simulink model "general_charger_2 (Jordans MacBook.lan's conflicted copy 2013-12-22)"  (R2013a)
settings: Solver=ode45  StartTime=0  StopTime=2.5  RelTol=1e-3
PreLoadFcn:
  | Ts =5e-6;
values from neighbouring files (symbols this model uses):
  ac_volt = 169    [charger_init.m]    (also in charger_init_simpl.m)
  Cdc = 2e-3    (= 0.002)    [charger_init.m]    (also in charger_init_simpl.m)
  dcAd = dcinvexp*(eye(dcnstates) + (Ts/2)*dcAc)    [charger_init.m]    (also in charger_init_simpl.m)
  dcBd = dcinvexp*dcBc    [charger_init.m]    (also in charger_init_simpl.m)
  dcCd = dcCc*dcinvexp*Ts    [charger_init.m]    (also in charger_init_simpl.m)
  dcDd = dcCc*dcinvexp*dcBc*(Ts/2) + dcDc    [charger_init.m]    (also in charger_init_simpl.m)
  Lin = 1.5e-3    (= 0.0015)    [charger_init.m]    (also in charger_init_simpl.m = 0.001)
  P = 1.92e3    (= 1920)    [charger_init.m]    (also in charger_init_simpl.m)
  Q = 0    [charger_init.m]    (also in charger_init_simpl.m)
  ramp = (dc_volt - Vdcmin)/(acdc_ramp_end_time)    (= 202)    [charger_init.m]    (also in charger_init_simpl.m = (dc_volt - Vdcmin)/(acdc_ramp_end_time))
  switch_Ts = 5e-5    (= 5e-05)    [charger_init.m]    (also in charger_init_simpl.m)
  sys_Ts = 5e-6    (= 5e-06)    [charger_init.m]    (also in charger_init_simpl.m)
  Vdcmin = ac_volt + 10    (= 179)    [charger_init.m]    (also in charger_init_simpl.m)
  voc = 105    [charger_init.m]    (also in charger_init_simpl.m)
undefined symbols (not defined in the file or in its folder): CESR, DiscIntNeverNeededParam, Rin
undefined symbols (not defined in the file): active_power_on, Ad, Bd, Cd, dc_volt, dcdc_iki, dcdc_ikp, dcdc_on, dcdc_vki, dcdc_vkp, Dd, dq_id_ki, dq_id_kp, dq_iq_ki, dq_iq_kp, dq_vdc_ki, dq_vdc_kp, P_ki, P_kp, Q_ki, Q_kp, reactive_power_on
libraries: simulink_extras x165, powerlib x52, simulink x29, powerlib_meascontrol x6
(part 2 of 6)

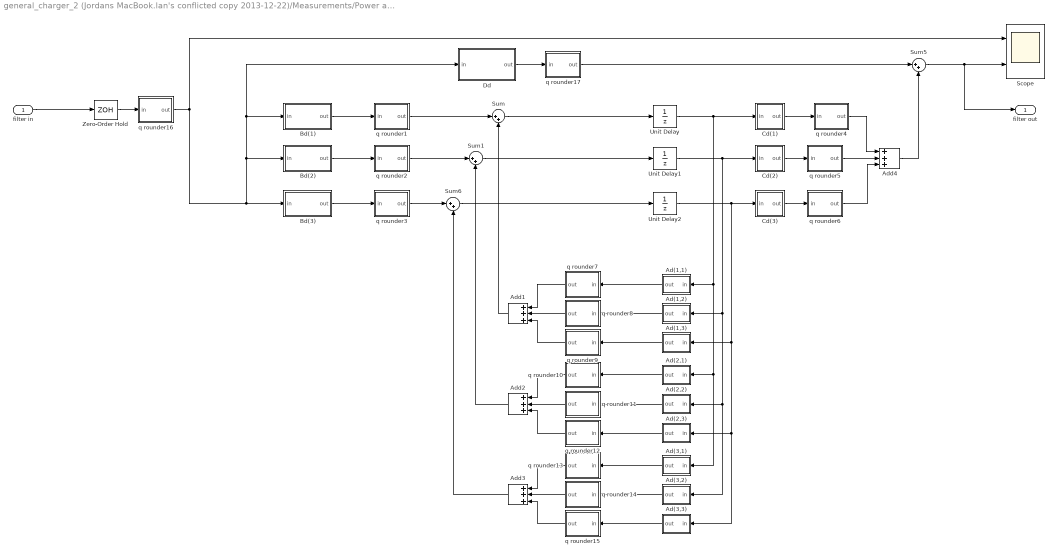
== system general_charger_2 (Jordans MacBook.lan's conflicted copy 2013-12-22)/Measurements/Power and angle calculations/discrete low pass filter1 ==
  filter in : Inport
  Ad(1,1) : Subsystem  mask{variable=Ad(1,1), nQ=29, maxRange=4}
      mask prompts: variable "state-space variable"; nQ "q value"; maxRange "max range"
      mask Display: disp(nQ)
  Ad(1,2) : Subsystem  mask{variable=Ad(1,2), nQ=23, maxRange=256}
      mask prompts: variable "state-space variable"; nQ "q value"; maxRange "max range"
      mask Display: disp(nQ)
  Ad(1,3) : Subsystem  mask{variable=Ad(1,3), nQ=14, maxRange=131072}
      mask prompts: variable "state-space variable"; nQ "q value"; maxRange "max range"
      mask Display: disp(nQ)
  Ad(2,1) : Subsystem  mask{variable=Ad(2,1), nQ=30, maxRange=2}
      mask prompts: variable "state-space variable"; nQ "q value"; maxRange "max range"
      mask Display: disp(nQ)
  Ad(2,2) : Subsystem  mask{variable=Ad(2,2), nQ=29, maxRange=4}
      mask prompts: variable "state-space variable"; nQ "q value"; maxRange "max range"
      mask Display: disp(nQ)
  Ad(2,3) : Subsystem  mask{variable=Ad(2,3), nQ=29, maxRange=4}
      mask prompts: variable "state-space variable"; nQ "q value"; maxRange "max range"
      mask Display: disp(nQ)
  Ad(3,1) : Subsystem  mask{variable=Ad(3,1), nQ=30, maxRange=2}
      mask prompts: variable "state-space variable"; nQ "q value"; maxRange "max range"
      mask Display: disp(nQ)
  Ad(3,2) : Subsystem  mask{variable=Ad(3,2), nQ=30, maxRange=2}
      mask prompts: variable "state-space variable"; nQ "q value"; maxRange "max range"
      mask Display: disp(nQ)
  Ad(3,3) : Subsystem  mask{variable=Ad(3,3), nQ=29, maxRange=4}
      mask prompts: variable "state-space variable"; nQ "q value"; maxRange "max range"
      mask Display: disp(nQ)
  Add{1..4} (4 alike) : Sum  Inputs=+++
  Bd(1) : Subsystem  mask{variable=Bd(1), nQ=29, maxRange=4}
      mask prompts: variable "state-space variable"; nQ "q value"; maxRange "max range"
      mask Display: disp(nQ)
  Bd(2) : Subsystem  mask{variable=Bd(2), nQ=30, maxRange=2}
      mask prompts: variable "state-space variable"; nQ "q value"; maxRange "max range"
      mask Display: disp(nQ)
  Bd(3) : Subsystem  mask{variable=Bd(3), nQ=30, maxRange=2}
      mask prompts: variable "state-space variable"; nQ "q value"; maxRange "max range"
      mask Display: disp(nQ)
  Cd(1) : Subsystem  mask{variable=Cd(1), nQ=30, maxRange=2}
      mask prompts: variable "state-space variable"; nQ "q value"; maxRange "max range"
      mask Display: disp(nQ)
  Cd(2) : Subsystem  mask{variable=Cd(2), nQ=23, maxRange=256}
      mask prompts: variable "state-space variable"; nQ "q value"; maxRange "max range"
      mask Display: disp(nQ)
  Cd(3) : Subsystem  mask{variable=Cd(3), nQ=15, maxRange=65536}
      mask prompts: variable "state-space variable"; nQ "q value"; maxRange "max range"
      mask Display: disp(nQ)
  Dd : Subsystem  mask{variable=Dd, nQ=30, maxRange=2}
      mask prompts: variable "state-space variable"; nQ "q value"; maxRange "max range"
      mask Display: disp(nQ)
  Scope : Scope  NumInputPorts=2
      settings: YMin=-5~-5  YMax=5~5  SaveName=ScopeData11
  Sum{,1,5..6} (4 alike) : Sum  Inputs=|++
  Unit Delay : UnitDelay  SampleTime=5e-5
  Unit Delay1 : UnitDelay  SampleTime=5e-5
  Unit Delay2 : UnitDelay  SampleTime=5e-5
  Zero-Order Hold : ZeroOrderHold  SampleTime=5e-5
  q rounder1 : Subsystem  mask{q=22, range=512}
      mask prompts: q "q value"; range "q range"
      mask Display: disp(q)
  q rounder10 : Subsystem  mask{q=30, range=2}
      mask prompts: q "q value"; range "q range"
      mask Display: disp(q)
  q rounder11 : Subsystem  mask{q=30, range=2}
      mask prompts: q "q value"; range "q range"
      mask Display: disp(q)
  q rounder12 : Subsystem  mask{q=30, range=2}
      mask prompts: q "q value"; range "q range"
      mask Display: disp(q)
  q rounder13 : Subsystem  mask{q=30, range=2}
      mask prompts: q "q value"; range "q range"
      mask Display: disp(q)
  q rounder14 : Subsystem  mask{q=30, range=2}
      mask prompts: q "q value"; range "q range"
      mask Display: disp(q)
  q rounder15 : Subsystem  mask{q=30, range=2}
      mask prompts: q "q value"; range "q range"
      mask Display: disp(q)
  q rounder16 : Subsystem  mask{q=19, range=4096}
      mask prompts: q "q value"; range "q range"
      mask Display: disp(q)
  q rounder17 : Subsystem  mask{q=30, range=2}
      mask prompts: q "q value"; range "q range"
      mask Display: disp(q)
  q rounder2 : Subsystem  mask{q=30, range=2}
      mask prompts: q "q value"; range "q range"
      mask Display: disp(q)
  q rounder3 : Subsystem  mask{q=30, range=2}
      mask prompts: q "q value"; range "q range"
      mask Display: disp(q)
  q rounder4 : Subsystem  mask{q=19, range=4096}
      mask prompts: q "q value"; range "q range"
      mask Display: disp(q)
  q rounder5 : Subsystem  mask{q=19, range=4096}
      mask prompts: q "q value"; range "q range"
      mask Display: disp(q)
  q rounder6 : Subsystem  mask{q=19, range=4096}
      mask prompts: q "q value"; range "q range"
      mask Display: disp(q)
  q rounder7 : Subsystem  mask{q=22, range=512}
      mask prompts: q "q value"; range "q range"
      mask Display: disp(q)
  q rounder8 : Subsystem  mask{q=22, range=512}
      mask prompts: q "q value"; range "q range"
      mask Display: disp(q)
  q rounder9 : Subsystem  mask{q=22, range=512}
      mask prompts: q "q value"; range "q range"
      mask Display: disp(q)
  filter out : Outport
  wires:
  Sum/1 -> Unit Delay/1
  Sum1/1 -> Unit Delay1/1
  Unit Delay/1 -> Ad(3,1)/1(in), Ad(2,1)/1(in), Ad(1,1)/1(in), Cd(1)/1(in)
  Unit Delay1/1 -> Ad(3,2)/1(in), Ad(2,2)/1(in), Ad(1,2)/1(in), Cd(2)/1(in)
  Dd/1(out) -> q rounder17/1(in)
  Sum5/1 -> filter out/1, Scope/2
  Zero-Order Hold/1 -> q rounder16/1(in)
  Sum6/1 -> Unit Delay2/1
  Unit Delay2/1 -> Ad(1,3)/1(in), Ad(3,3)/1(in), Ad(2,3)/1(in), Cd(3)/1(in)
  Ad(1,2)/1(out) -> q rounder8/1(in)
  Ad(1,1)/1(out) -> q rounder7/1(in)
  Ad(2,1)/1(out) -> q rounder10/1(in)
  Ad(2,3)/1(out) -> q rounder12/1(in)
  Ad(2,2)/1(out) -> q rounder11/1(in)
  Ad(3,2)/1(out) -> q rounder14/1(in)
  Ad(3,1)/1(out) -> q rounder13/1(in)
  Ad(3,3)/1(out) -> q rounder15/1(in)
  Add2/1 -> Sum1/2
  Add3/1 -> Sum6/2
  q rounder2/1(out) -> Sum1/1
  q rounder3/1(out) -> Sum6/1
  q rounder4/1(out) -> Add4/1
  q rounder5/1(out) -> Add4/2
  q rounder6/1(out) -> Add4/3
  q rounder7/1(out) -> Add1/1
  q rounder8/1(out) -> Add1/2
  q rounder9/1(out) -> Add1/3
  q rounder10/1(out) -> Add2/1
  q rounder11/1(out) -> Add2/2
  q rounder12/1(out) -> Add2/3
  q rounder13/1(out) -> Add3/1
  q rounder14/1(out) -> Add3/2
  q rounder15/1(out) -> Add3/3
  Bd(1)/1(out) -> q rounder1/1(in)
  Cd(1)/1(out) -> q rounder4/1(in)
  Bd(2)/1(out) -> q rounder2/1(in)
  Bd(3)/1(out) -> q rounder3/1(in)
  Cd(3)/1(out) -> q rounder6/1(in)
  Cd(2)/1(out) -> q rounder5/1(in)
  Ad(1,3)/1(out) -> q rounder9/1(in)
  q rounder16/1(out) -> Scope/1, Bd(3)/1(in), Bd(2)/1(in), Dd/1(in), Bd(1)/1(in)
  q rounder17/1(out) -> Sum5/1
  Add4/1 -> Sum5/2
  Add1/1 -> Sum/2
  q rounder1/1(out) -> Sum/1
  filter in/1 -> Zero-Order Hold/1

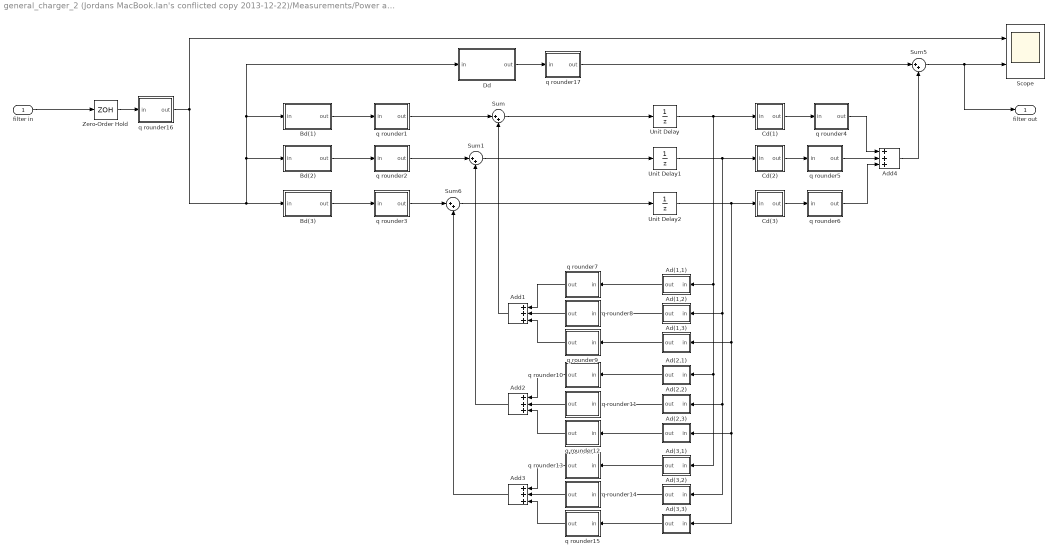
== system general_charger_2 (Jordans MacBook.lan's conflicted copy 2013-12-22)/Measurements/Power and angle calculations/discrete low pass filter2 ==
  filter in : Inport
  Ad(1,1) : Subsystem  mask{variable=Ad(1,1), nQ=29, maxRange=4}
      mask prompts: variable "state-space variable"; nQ "q value"; maxRange "max range"
      mask Display: disp(nQ)
  Ad(1,2) : Subsystem  mask{variable=Ad(1,2), nQ=23, maxRange=256}
      mask prompts: variable "state-space variable"; nQ "q value"; maxRange "max range"
      mask Display: disp(nQ)
  Ad(1,3) : Subsystem  mask{variable=Ad(1,3), nQ=14, maxRange=131072}
      mask prompts: variable "state-space variable"; nQ "q value"; maxRange "max range"
      mask Display: disp(nQ)
  Ad(2,1) : Subsystem  mask{variable=Ad(2,1), nQ=30, maxRange=2}
      mask prompts: variable "state-space variable"; nQ "q value"; maxRange "max range"
      mask Display: disp(nQ)
  Ad(2,2) : Subsystem  mask{variable=Ad(2,2), nQ=29, maxRange=4}
      mask prompts: variable "state-space variable"; nQ "q value"; maxRange "max range"
      mask Display: disp(nQ)
  Ad(2,3) : Subsystem  mask{variable=Ad(2,3), nQ=29, maxRange=4}
      mask prompts: variable "state-space variable"; nQ "q value"; maxRange "max range"
      mask Display: disp(nQ)
  Ad(3,1) : Subsystem  mask{variable=Ad(3,1), nQ=30, maxRange=2}
      mask prompts: variable "state-space variable"; nQ "q value"; maxRange "max range"
      mask Display: disp(nQ)
  Ad(3,2) : Subsystem  mask{variable=Ad(3,2), nQ=30, maxRange=2}
      mask prompts: variable "state-space variable"; nQ "q value"; maxRange "max range"
      mask Display: disp(nQ)
  Ad(3,3) : Subsystem  mask{variable=Ad(3,3), nQ=29, maxRange=4}
      mask prompts: variable "state-space variable"; nQ "q value"; maxRange "max range"
      mask Display: disp(nQ)
  Add{1..4} (4 alike) : Sum  Inputs=+++
  Bd(1) : Subsystem  mask{variable=Bd(1), nQ=29, maxRange=4}
      mask prompts: variable "state-space variable"; nQ "q value"; maxRange "max range"
      mask Display: disp(nQ)
  Bd(2) : Subsystem  mask{variable=Bd(2), nQ=30, maxRange=2}
      mask prompts: variable "state-space variable"; nQ "q value"; maxRange "max range"
      mask Display: disp(nQ)
  Bd(3) : Subsystem  mask{variable=Bd(3), nQ=30, maxRange=2}
      mask prompts: variable "state-space variable"; nQ "q value"; maxRange "max range"
      mask Display: disp(nQ)
  Cd(1) : Subsystem  mask{variable=Cd(1), nQ=30, maxRange=2}
      mask prompts: variable "state-space variable"; nQ "q value"; maxRange "max range"
      mask Display: disp(nQ)
  Cd(2) : Subsystem  mask{variable=Cd(2), nQ=23, maxRange=256}
      mask prompts: variable "state-space variable"; nQ "q value"; maxRange "max range"
      mask Display: disp(nQ)
  Cd(3) : Subsystem  mask{variable=Cd(3), nQ=15, maxRange=65536}
      mask prompts: variable "state-space variable"; nQ "q value"; maxRange "max range"
      mask Display: disp(nQ)
  Dd : Subsystem  mask{variable=Dd, nQ=30, maxRange=2}
      mask prompts: variable "state-space variable"; nQ "q value"; maxRange "max range"
      mask Display: disp(nQ)
  Scope : Scope  NumInputPorts=2
      settings: YMin=-5~-5  YMax=5~5  SaveName=ScopeData11
  Sum{,1,5..6} (4 alike) : Sum  Inputs=|++
  Unit Delay : UnitDelay  SampleTime=5e-5
  Unit Delay1 : UnitDelay  SampleTime=5e-5
  Unit Delay2 : UnitDelay  SampleTime=5e-5
  Zero-Order Hold : ZeroOrderHold  SampleTime=5e-5
  q rounder1 : Subsystem  mask{q=22, range=512}
      mask prompts: q "q value"; range "q range"
      mask Display: disp(q)
  q rounder10 : Subsystem  mask{q=30, range=2}
      mask prompts: q "q value"; range "q range"
      mask Display: disp(q)
  q rounder11 : Subsystem  mask{q=30, range=2}
      mask prompts: q "q value"; range "q range"
      mask Display: disp(q)
  q rounder12 : Subsystem  mask{q=30, range=2}
      mask prompts: q "q value"; range "q range"
      mask Display: disp(q)
  q rounder13 : Subsystem  mask{q=30, range=2}
      mask prompts: q "q value"; range "q range"
      mask Display: disp(q)
  q rounder14 : Subsystem  mask{q=30, range=2}
      mask prompts: q "q value"; range "q range"
      mask Display: disp(q)
  q rounder15 : Subsystem  mask{q=30, range=2}
      mask prompts: q "q value"; range "q range"
      mask Display: disp(q)
  q rounder16 : Subsystem  mask{q=19, range=4096}
      mask prompts: q "q value"; range "q range"
      mask Display: disp(q)
  q rounder17 : Subsystem  mask{q=30, range=2}
      mask prompts: q "q value"; range "q range"
      mask Display: disp(q)
  q rounder2 : Subsystem  mask{q=30, range=2}
      mask prompts: q "q value"; range "q range"
      mask Display: disp(q)
  q rounder3 : Subsystem  mask{q=30, range=2}
      mask prompts: q "q value"; range "q range"
      mask Display: disp(q)
  q rounder4 : Subsystem  mask{q=19, range=4096}
      mask prompts: q "q value"; range "q range"
      mask Display: disp(q)
  q rounder5 : Subsystem  mask{q=19, range=4096}
      mask prompts: q "q value"; range "q range"
      mask Display: disp(q)
  q rounder6 : Subsystem  mask{q=19, range=4096}
      mask prompts: q "q value"; range "q range"
      mask Display: disp(q)
  q rounder7 : Subsystem  mask{q=22, range=512}
      mask prompts: q "q value"; range "q range"
      mask Display: disp(q)
  q rounder8 : Subsystem  mask{q=22, range=512}
      mask prompts: q "q value"; range "q range"
      mask Display: disp(q)
  q rounder9 : Subsystem  mask{q=22, range=512}
      mask prompts: q "q value"; range "q range"
      mask Display: disp(q)
  filter out : Outport
  wires:
  Sum/1 -> Unit Delay/1
  Sum1/1 -> Unit Delay1/1
  Unit Delay/1 -> Ad(3,1)/1(in), Ad(2,1)/1(in), Ad(1,1)/1(in), Cd(1)/1(in)
  Unit Delay1/1 -> Ad(3,2)/1(in), Ad(2,2)/1(in), Ad(1,2)/1(in), Cd(2)/1(in)
  Dd/1(out) -> q rounder17/1(in)
  Sum5/1 -> filter out/1, Scope/2
  Zero-Order Hold/1 -> q rounder16/1(in)
  Sum6/1 -> Unit Delay2/1
  Unit Delay2/1 -> Ad(1,3)/1(in), Ad(3,3)/1(in), Ad(2,3)/1(in), Cd(3)/1(in)
  Ad(1,2)/1(out) -> q rounder8/1(in)
  Ad(1,1)/1(out) -> q rounder7/1(in)
  Ad(2,1)/1(out) -> q rounder10/1(in)
  Ad(2,3)/1(out) -> q rounder12/1(in)
  Ad(2,2)/1(out) -> q rounder11/1(in)
  Ad(3,2)/1(out) -> q rounder14/1(in)
  Ad(3,1)/1(out) -> q rounder13/1(in)
  Ad(3,3)/1(out) -> q rounder15/1(in)
  Add2/1 -> Sum1/2
  Add3/1 -> Sum6/2
  q rounder2/1(out) -> Sum1/1
  q rounder3/1(out) -> Sum6/1
  q rounder4/1(out) -> Add4/1
  q rounder5/1(out) -> Add4/2
  q rounder6/1(out) -> Add4/3
  q rounder7/1(out) -> Add1/1
  q rounder8/1(out) -> Add1/2
  q rounder9/1(out) -> Add1/3
  q rounder10/1(out) -> Add2/1
  q rounder11/1(out) -> Add2/2
  q rounder12/1(out) -> Add2/3
  q rounder13/1(out) -> Add3/1
  q rounder14/1(out) -> Add3/2
  q rounder15/1(out) -> Add3/3
  Bd(1)/1(out) -> q rounder1/1(in)
  Cd(1)/1(out) -> q rounder4/1(in)
  Bd(2)/1(out) -> q rounder2/1(in)
  Bd(3)/1(out) -> q rounder3/1(in)
  Cd(3)/1(out) -> q rounder6/1(in)
  Cd(2)/1(out) -> q rounder5/1(in)
  Ad(1,3)/1(out) -> q rounder9/1(in)
  q rounder16/1(out) -> Scope/1, Bd(3)/1(in), Bd(2)/1(in), Dd/1(in), Bd(1)/1(in)
  q rounder17/1(out) -> Sum5/1
  Add4/1 -> Sum5/2
  Add1/1 -> Sum/2
  q rounder1/1(out) -> Sum/1
  filter in/1 -> Zero-Order Hold/1

== system general_charger_2 (Jordans MacBook.lan's conflicted copy 2013-12-22)/Measurements/THD/RMS1 ==
  ac in : Inport
  Constant1 : Constant  Value=f  SampleTime=Tsss
  Constant2 : Constant  Value=K1  SampleTime=Tsss
  Constant3 : Constant  Value=K2  SampleTime=Tsss
  Delay : Delay  DelayLength=ceil(SpC)  SampleTime=Tsss
  Gain : Gain  Gain=K1  SaturateOnIntegerOverflow=on  OutDataTypeStr=Inherit: Same as input  ParamDataTypeStr=Inherit: Same as input
  Gain1 : Gain  Gain=K2  SaturateOnIntegerOverflow=on  OutDataTypeStr=Inherit: Same as input  ParamDataTypeStr=Inherit: Same as input
  PI3 : Subsystem  mask{ki=1, kp=0, Ts_pi=5e-5, int_sat_up=inf, int_sat_low=-inf, pi_sat_up=inf, pi_sat_low=-inf}
      mask prompts: ki "Integral Gain"; kp "Proportional Gain"; Ts_pi "Sample Time"; int_sat_up "Integral Saturation Upper"; int_sat_low "Integral Saturation Lower"; pi_sat_up "PI Controller Saturation Upper"; pi_sat_low "PI Controller Saturation Lower"
      mask Display: disp('PI')
  Product3 : Product  SaturateOnIntegerOverflow=on  InputSameDT=on  OutDataTypeStr=Inherit: Same as first input
  Product4 : Product  SaturateOnIntegerOverflow=on  InputSameDT=on  OutDataTypeStr=Inherit: Same as first input
  Saturation : Saturate  UpperLimit=inf  LowerLimit=0
  Scope1 : Scope  NumInputPorts=3
      settings: ShowLegends=on  TimeRange=1  YMin=0~-5~-5  YMax=32.5~5~5  SaveName=is_vs_7  MaxDataPoints=50000
  Scope2 : Scope  NumInputPorts=3
      settings: ShowLegends=on  TimeRange=1  YMin=0~-5~-5  YMax=32.5~5~5  SaveName=is_vs_  MaxDataPoints=50000
  Scope3 : Scope  NumInputPorts=3
      settings: ShowLegends=on  TimeRange=1  YMin=0~-5~-5  YMax=32.5~5~5  SaveName=is_vs_8  MaxDataPoints=50000
  Sqrt : Sqrt  SaturateOnIntegerOverflow=on
  Sum1 : Sum  Inputs=+-  SaturateOnIntegerOverflow=on  InputSameDT=on  OutDataTypeStr=Inherit: Same as first input
  Sum2 : Sum  Inputs=-+  SaturateOnIntegerOverflow=on  InputSameDT=on  OutDataTypeStr=Inherit: Same as first input
  Sum3 : Sum  SaturateOnIntegerOverflow=on  InputSameDT=on  OutDataTypeStr=Inherit: Same as first input
  Unit Delay : UnitDelay  SampleTime=Tsss
  rms out : Outport
  wires:
  Sum2/1 -> Product4/1
  Constant1/1 -> Product4/2
  Delay/1 -> Scope1/2, Sum2/1
  ac in/1 -> Product3/2, Product3/1
  Product3/1 -> Gain1/1, Unit Delay/1, PI3/1(in)
  PI3/1(out) -> Scope1/1, Sum2/2, Delay/1
  Sqrt/1 -> rms out/1
  Gain1/1 -> Scope2/1, Sum1/1
  Unit Delay/1 -> Gain/1
  Gain/1 -> Scope2/2, Sum1/2
  Product4/1 -> Sum3/1
  Sum3/1 -> Saturation/1
  Sum1/1 -> Scope2/3, Sum3/2  "Correction"
  Saturation/1 -> Sqrt/1
  Constant2/1 -> Scope3/1
  Constant3/1 -> Scope3/2

== system general_charger_2 (Jordans MacBook.lan's conflicted copy 2013-12-22)/Measurements/THD/RMS2 ==
  ac in : Inport
  Constant1 : Constant  Value=f  SampleTime=Tsss
  Constant2 : Constant  Value=K1  SampleTime=Tsss
  Constant3 : Constant  Value=K2  SampleTime=Tsss
  Delay : Delay  DelayLength=ceil(SpC)  SampleTime=Tsss
  Gain : Gain  Gain=K1  SaturateOnIntegerOverflow=on  OutDataTypeStr=Inherit: Same as input  ParamDataTypeStr=Inherit: Same as input
  Gain1 : Gain  Gain=K2  SaturateOnIntegerOverflow=on  OutDataTypeStr=Inherit: Same as input  ParamDataTypeStr=Inherit: Same as input
  PI3 : Subsystem  mask{ki=1, kp=0, Ts_pi=5e-5, int_sat_up=inf, int_sat_low=-inf, pi_sat_up=inf, pi_sat_low=-inf}
      mask prompts: ki "Integral Gain"; kp "Proportional Gain"; Ts_pi "Sample Time"; int_sat_up "Integral Saturation Upper"; int_sat_low "Integral Saturation Lower"; pi_sat_up "PI Controller Saturation Upper"; pi_sat_low "PI Controller Saturation Lower"
      mask Display: disp('PI')
  Product3 : Product  SaturateOnIntegerOverflow=on  InputSameDT=on  OutDataTypeStr=Inherit: Same as first input
  Product4 : Product  SaturateOnIntegerOverflow=on  InputSameDT=on  OutDataTypeStr=Inherit: Same as first input
  Saturation : Saturate  UpperLimit=inf  LowerLimit=0
  Scope1 : Scope  NumInputPorts=3
      settings: ShowLegends=on  TimeRange=1  YMin=0~-5~-5  YMax=32.5~5~5  SaveName=is_vs_7  MaxDataPoints=50000
  Scope2 : Scope  NumInputPorts=3
      settings: ShowLegends=on  TimeRange=1  YMin=0~-5~-5  YMax=32.5~5~5  SaveName=is_vs_  MaxDataPoints=50000
  Scope3 : Scope  NumInputPorts=3
      settings: ShowLegends=on  TimeRange=1  YMin=0~-5~-5  YMax=32.5~5~5  SaveName=is_vs_8  MaxDataPoints=50000
  Sqrt : Sqrt  SaturateOnIntegerOverflow=on
  Sum1 : Sum  Inputs=+-  SaturateOnIntegerOverflow=on  InputSameDT=on  OutDataTypeStr=Inherit: Same as first input
  Sum2 : Sum  Inputs=-+  SaturateOnIntegerOverflow=on  InputSameDT=on  OutDataTypeStr=Inherit: Same as first input
  Sum3 : Sum  SaturateOnIntegerOverflow=on  InputSameDT=on  OutDataTypeStr=Inherit: Same as first input
  Unit Delay : UnitDelay  SampleTime=Tsss
  rms out : Outport
  wires:
  Sum2/1 -> Product4/1
  Constant1/1 -> Product4/2
  Delay/1 -> Scope1/2, Sum2/1
  ac in/1 -> Product3/2, Product3/1
  Product3/1 -> Gain1/1, Unit Delay/1, PI3/1(in)
  PI3/1(out) -> Scope1/1, Sum2/2, Delay/1
  Sqrt/1 -> rms out/1
  Gain1/1 -> Scope2/1, Sum1/1
  Unit Delay/1 -> Gain/1
  Gain/1 -> Scope2/2, Sum1/2
  Product4/1 -> Sum3/1
  Sum3/1 -> Saturation/1
  Sum1/1 -> Scope2/3, Sum3/2  "Correction"
  Saturation/1 -> Sqrt/1
  Constant2/1 -> Scope3/1
  Constant3/1 -> Scope3/2

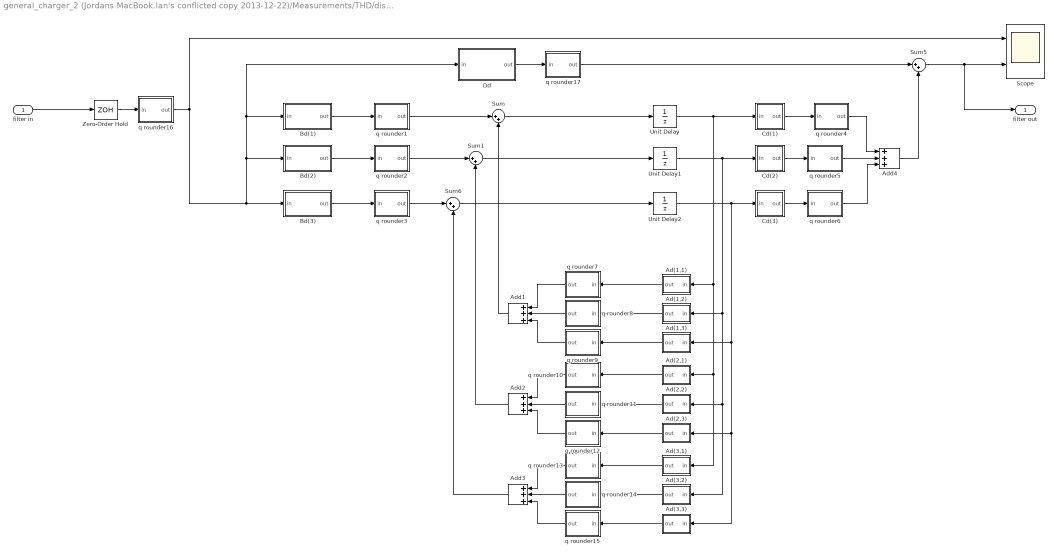
== system general_charger_2 (Jordans MacBook.lan's conflicted copy 2013-12-22)/Measurements/THD/discrete low pass filter1 ==
  filter in : Inport
  Ad(1,1) : Subsystem  mask{variable=Ad(1,1), nQ=29, maxRange=4}
      mask prompts: variable "state-space variable"; nQ "q value"; maxRange "max range"
      mask Display: disp(nQ)
  Ad(1,2) : Subsystem  mask{variable=Ad(1,2), nQ=23, maxRange=256}
      mask prompts: variable "state-space variable"; nQ "q value"; maxRange "max range"
      mask Display: disp(nQ)
  Ad(1,3) : Subsystem  mask{variable=Ad(1,3), nQ=14, maxRange=131072}
      mask prompts: variable "state-space variable"; nQ "q value"; maxRange "max range"
      mask Display: disp(nQ)
  Ad(2,1) : Subsystem  mask{variable=Ad(2,1), nQ=30, maxRange=2}
      mask prompts: variable "state-space variable"; nQ "q value"; maxRange "max range"
      mask Display: disp(nQ)
  Ad(2,2) : Subsystem  mask{variable=Ad(2,2), nQ=29, maxRange=4}
      mask prompts: variable "state-space variable"; nQ "q value"; maxRange "max range"
      mask Display: disp(nQ)
  Ad(2,3) : Subsystem  mask{variable=Ad(2,3), nQ=29, maxRange=4}
      mask prompts: variable "state-space variable"; nQ "q value"; maxRange "max range"
      mask Display: disp(nQ)
  Ad(3,1) : Subsystem  mask{variable=Ad(3,1), nQ=30, maxRange=2}
      mask prompts: variable "state-space variable"; nQ "q value"; maxRange "max range"
      mask Display: disp(nQ)
  Ad(3,2) : Subsystem  mask{variable=Ad(3,2), nQ=30, maxRange=2}
      mask prompts: variable "state-space variable"; nQ "q value"; maxRange "max range"
      mask Display: disp(nQ)
  Ad(3,3) : Subsystem  mask{variable=Ad(3,3), nQ=29, maxRange=4}
      mask prompts: variable "state-space variable"; nQ "q value"; maxRange "max range"
      mask Display: disp(nQ)
  Add{1..4} (4 alike) : Sum  Inputs=+++
  Bd(1) : Subsystem  mask{variable=Bd(1), nQ=29, maxRange=4}
      mask prompts: variable "state-space variable"; nQ "q value"; maxRange "max range"
      mask Display: disp(nQ)
  Bd(2) : Subsystem  mask{variable=Bd(2), nQ=30, maxRange=2}
      mask prompts: variable "state-space variable"; nQ "q value"; maxRange "max range"
      mask Display: disp(nQ)
  Bd(3) : Subsystem  mask{variable=Bd(3), nQ=30, maxRange=2}
      mask prompts: variable "state-space variable"; nQ "q value"; maxRange "max range"
      mask Display: disp(nQ)
  Cd(1) : Subsystem  mask{variable=Cd(1), nQ=30, maxRange=2}
      mask prompts: variable "state-space variable"; nQ "q value"; maxRange "max range"
      mask Display: disp(nQ)
  Cd(2) : Subsystem  mask{variable=Cd(2), nQ=23, maxRange=256}
      mask prompts: variable "state-space variable"; nQ "q value"; maxRange "max range"
      mask Display: disp(nQ)
  Cd(3) : Subsystem  mask{variable=Cd(3), nQ=15, maxRange=65536}
      mask prompts: variable "state-space variable"; nQ "q value"; maxRange "max range"
      mask Display: disp(nQ)
  Dd : Subsystem  mask{variable=Dd, nQ=30, maxRange=2}
      mask prompts: variable "state-space variable"; nQ "q value"; maxRange "max range"
      mask Display: disp(nQ)
  Scope : Scope  NumInputPorts=2
      settings: YMin=-5~-5  YMax=5~5  SaveName=ScopeData11
  Sum{,1,5..6} (4 alike) : Sum  Inputs=|++
  Unit Delay : UnitDelay  SampleTime=5e-5
  Unit Delay1 : UnitDelay  SampleTime=5e-5
  Unit Delay2 : UnitDelay  SampleTime=5e-5
  Zero-Order Hold : ZeroOrderHold  SampleTime=5e-5
  q rounder1 : Subsystem  mask{q=22, range=512}
      mask prompts: q "q value"; range "q range"
      mask Display: disp(q)
  q rounder10 : Subsystem  mask{q=30, range=2}
      mask prompts: q "q value"; range "q range"
      mask Display: disp(q)
  q rounder11 : Subsystem  mask{q=30, range=2}
      mask prompts: q "q value"; range "q range"
      mask Display: disp(q)
  q rounder12 : Subsystem  mask{q=30, range=2}
      mask prompts: q "q value"; range "q range"
      mask Display: disp(q)
  q rounder13 : Subsystem  mask{q=30, range=2}
      mask prompts: q "q value"; range "q range"
      mask Display: disp(q)
  q rounder14 : Subsystem  mask{q=30, range=2}
      mask prompts: q "q value"; range "q range"
      mask Display: disp(q)
  q rounder15 : Subsystem  mask{q=30, range=2}
      mask prompts: q "q value"; range "q range"
      mask Display: disp(q)
  q rounder16 : Subsystem  mask{q=19, range=4096}
      mask prompts: q "q value"; range "q range"
      mask Display: disp(q)
  q rounder17 : Subsystem  mask{q=30, range=2}
      mask prompts: q "q value"; range "q range"
      mask Display: disp(q)
  q rounder2 : Subsystem  mask{q=30, range=2}
      mask prompts: q "q value"; range "q range"
      mask Display: disp(q)
  q rounder3 : Subsystem  mask{q=30, range=2}
      mask prompts: q "q value"; range "q range"
      mask Display: disp(q)
  q rounder4 : Subsystem  mask{q=19, range=4096}
      mask prompts: q "q value"; range "q range"
      mask Display: disp(q)
  q rounder5 : Subsystem  mask{q=19, range=4096}
      mask prompts: q "q value"; range "q range"
      mask Display: disp(q)
  q rounder6 : Subsystem  mask{q=19, range=4096}
      mask prompts: q "q value"; range "q range"
      mask Display: disp(q)
  q rounder7 : Subsystem  mask{q=22, range=512}
      mask prompts: q "q value"; range "q range"
      mask Display: disp(q)
  q rounder8 : Subsystem  mask{q=22, range=512}
      mask prompts: q "q value"; range "q range"
      mask Display: disp(q)
  q rounder9 : Subsystem  mask{q=22, range=512}
      mask prompts: q "q value"; range "q range"
      mask Display: disp(q)
  filter out : Outport
  wires:
  Sum/1 -> Unit Delay/1
  Sum1/1 -> Unit Delay1/1
  Unit Delay/1 -> Ad(3,1)/1(in), Ad(2,1)/1(in), Ad(1,1)/1(in), Cd(1)/1(in)
  Unit Delay1/1 -> Ad(3,2)/1(in), Ad(2,2)/1(in), Ad(1,2)/1(in), Cd(2)/1(in)
  Dd/1(out) -> q rounder17/1(in)
  Sum5/1 -> filter out/1, Scope/2
  Zero-Order Hold/1 -> q rounder16/1(in)
  Sum6/1 -> Unit Delay2/1
  Unit Delay2/1 -> Ad(1,3)/1(in), Ad(3,3)/1(in), Ad(2,3)/1(in), Cd(3)/1(in)
  Ad(1,2)/1(out) -> q rounder8/1(in)
  Ad(1,1)/1(out) -> q rounder7/1(in)
  Ad(2,1)/1(out) -> q rounder10/1(in)
  Ad(2,3)/1(out) -> q rounder12/1(in)
  Ad(2,2)/1(out) -> q rounder11/1(in)
  Ad(3,2)/1(out) -> q rounder14/1(in)
  Ad(3,1)/1(out) -> q rounder13/1(in)
  Ad(3,3)/1(out) -> q rounder15/1(in)
  Add2/1 -> Sum1/2
  Add3/1 -> Sum6/2
  q rounder2/1(out) -> Sum1/1
  q rounder3/1(out) -> Sum6/1
  q rounder4/1(out) -> Add4/1
  q rounder5/1(out) -> Add4/2
  q rounder6/1(out) -> Add4/3
  q rounder7/1(out) -> Add1/1
  q rounder8/1(out) -> Add1/2
  q rounder9/1(out) -> Add1/3
  q rounder10/1(out) -> Add2/1
  q rounder11/1(out) -> Add2/2
  q rounder12/1(out) -> Add2/3
  q rounder13/1(out) -> Add3/1
  q rounder14/1(out) -> Add3/2
  q rounder15/1(out) -> Add3/3
  Bd(1)/1(out) -> q rounder1/1(in)
  Cd(1)/1(out) -> q rounder4/1(in)
  Bd(2)/1(out) -> q rounder2/1(in)
  Bd(3)/1(out) -> q rounder3/1(in)
  Cd(3)/1(out) -> q rounder6/1(in)
  Cd(2)/1(out) -> q rounder5/1(in)
  Ad(1,3)/1(out) -> q rounder9/1(in)
  q rounder16/1(out) -> Scope/1, Bd(3)/1(in), Bd(2)/1(in), Dd/1(in), Bd(1)/1(in)
  q rounder17/1(out) -> Sum5/1
  Add4/1 -> Sum5/2
  Add1/1 -> Sum/2
  q rounder1/1(out) -> Sum/1
  filter in/1 -> Zero-Order Hold/1

== system general_charger_2 (Jordans MacBook.lan's conflicted copy 2013-12-22)/Measurements/discrete low pass filter1/Ad(1,1) ==
  in : Inport
  Constant1 : Constant  Value=variable
  Product1 : Product
  q rounder16 : Subsystem  mask{q=nQ, range=maxRange}
      mask prompts: q "q value"; range "q range"
  out : Outport
  wires:
  q rounder16/1(out) -> Product1/1
  Constant1/1 -> q rounder16/1(in)
  Product1/1 -> out/1
  in/1 -> Product1/2

== system general_charger_2 (Jordans MacBook.lan's conflicted copy 2013-12-22)/Measurements/discrete low pass filter1/Ad(1,2) ==
  in : Inport
  Constant1 : Constant  Value=variable
  Product1 : Product
  q rounder16 : Subsystem  mask{q=nQ, range=maxRange}
      mask prompts: q "q value"; range "q range"
  out : Outport
  wires:
  q rounder16/1(out) -> Product1/1
  Constant1/1 -> q rounder16/1(in)
  Product1/1 -> out/1
  in/1 -> Product1/2

== system general_charger_2 (Jordans MacBook.lan's conflicted copy 2013-12-22)/Measurements/discrete low pass filter1/Ad(1,3) ==
  in : Inport
  Constant1 : Constant  Value=variable
  Product1 : Product
  Scope1 : Scope  NumInputPorts=2
      settings: YMin=-5~-5  YMax=5~5
  q rounder16 : Subsystem  mask{q=nQ, range=maxRange}
      mask prompts: q "q value"; range "q range"
  out : Outport
  wires:
  q rounder16/1(out) -> Product1/1, Scope1/2
  Constant1/1 -> Scope1/1, q rounder16/1(in)
  Product1/1 -> out/1
  in/1 -> Product1/2

== system general_charger_2 (Jordans MacBook.lan's conflicted copy 2013-12-22)/Measurements/discrete low pass filter1/Ad(2,1) ==
  in : Inport
  Constant1 : Constant  Value=variable
  Product1 : Product
  Scope1 : Scope  NumInputPorts=2
      settings: YMin=-5~-5  YMax=5~5
  q rounder16 : Subsystem  mask{q=nQ, range=maxRange}
      mask prompts: q "q value"; range "q range"
  out : Outport
  wires:
  q rounder16/1(out) -> Product1/1, Scope1/2
  Constant1/1 -> Scope1/1, q rounder16/1(in)
  Product1/1 -> out/1
  in/1 -> Product1/2

== system general_charger_2 (Jordans MacBook.lan's conflicted copy 2013-12-22)/Measurements/discrete low pass filter1/Ad(2,2) ==
  in : Inport
  Constant1 : Constant  Value=variable
  Product1 : Product
  Scope1 : Scope  NumInputPorts=2
      settings: YMin=-5~-5  YMax=5~5
  q rounder16 : Subsystem  mask{q=nQ, range=maxRange}
      mask prompts: q "q value"; range "q range"
  out : Outport
  wires:
  q rounder16/1(out) -> Product1/1, Scope1/2
  Constant1/1 -> Scope1/1, q rounder16/1(in)
  Product1/1 -> out/1
  in/1 -> Product1/2

== system general_charger_2 (Jordans MacBook.lan's conflicted copy 2013-12-22)/Measurements/discrete low pass filter1/Ad(2,3) ==
  in : Inport
  Constant1 : Constant  Value=variable
  Product1 : Product
  Scope1 : Scope  NumInputPorts=2
      settings: YMin=-5~-5  YMax=5~5
  q rounder16 : Subsystem  mask{q=nQ, range=maxRange}
      mask prompts: q "q value"; range "q range"
  out : Outport
  wires:
  q rounder16/1(out) -> Product1/1, Scope1/2
  Constant1/1 -> Scope1/1, q rounder16/1(in)
  Product1/1 -> out/1
  in/1 -> Product1/2

== system general_charger_2 (Jordans MacBook.lan's conflicted copy 2013-12-22)/Measurements/discrete low pass filter1/Ad(3,1) ==
  in : Inport
  Constant1 : Constant  Value=variable
  Product1 : Product
  Scope1 : Scope  NumInputPorts=2
      settings: YMin=-5~-5  YMax=5~5
  q rounder16 : Subsystem  mask{q=nQ, range=maxRange}
      mask prompts: q "q value"; range "q range"
  out : Outport
  wires:
  q rounder16/1(out) -> Product1/1, Scope1/2
  Constant1/1 -> Scope1/1, q rounder16/1(in)
  Product1/1 -> out/1
  in/1 -> Product1/2

== system general_charger_2 (Jordans MacBook.lan's conflicted copy 2013-12-22)/Measurements/discrete low pass filter1/Ad(3,2) ==
  in : Inport
  Constant1 : Constant  Value=variable
  Product1 : Product
  Scope1 : Scope  NumInputPorts=2
      settings: YMin=-5~-5  YMax=5~5
  q rounder16 : Subsystem  mask{q=nQ, range=maxRange}
      mask prompts: q "q value"; range "q range"
  out : Outport
  wires:
  q rounder16/1(out) -> Product1/1, Scope1/2
  Constant1/1 -> Scope1/1, q rounder16/1(in)
  Product1/1 -> out/1
  in/1 -> Product1/2

== system general_charger_2 (Jordans MacBook.lan's conflicted copy 2013-12-22)/Measurements/discrete low pass filter1/Ad(3,3) ==
  in : Inport
  Constant1 : Constant  Value=variable
  Product1 : Product
  Scope1 : Scope  NumInputPorts=2
      settings: YMin=-5~-5  YMax=5~5
  q rounder16 : Subsystem  mask{q=nQ, range=maxRange}
      mask prompts: q "q value"; range "q range"
  out : Outport
  wires:
  q rounder16/1(out) -> Product1/1, Scope1/2
  Constant1/1 -> Scope1/1, q rounder16/1(in)
  Product1/1 -> out/1
  in/1 -> Product1/2

== system general_charger_2 (Jordans MacBook.lan's conflicted copy 2013-12-22)/Measurements/discrete low pass filter1/Bd(1) ==
  in : Inport
  Constant1 : Constant  Value=variable
  Product1 : Product
  q rounder16 : Subsystem  mask{q=nQ, range=maxRange}
      mask prompts: q "q value"; range "q range"
  out : Outport
  wires:
  q rounder16/1(out) -> Product1/1
  Constant1/1 -> q rounder16/1(in)
  Product1/1 -> out/1
  in/1 -> Product1/2

== system general_charger_2 (Jordans MacBook.lan's conflicted copy 2013-12-22)/Measurements/discrete low pass filter1/Bd(2) ==
  in : Inport
  Constant1 : Constant  Value=variable
  Product1 : Product
  q rounder16 : Subsystem  mask{q=nQ, range=maxRange}
      mask prompts: q "q value"; range "q range"
  out : Outport
  wires:
  q rounder16/1(out) -> Product1/1
  Constant1/1 -> q rounder16/1(in)
  Product1/1 -> out/1
  in/1 -> Product1/2

== system general_charger_2 (Jordans MacBook.lan's conflicted copy 2013-12-22)/Measurements/discrete low pass filter1/Bd(3) ==
  in : Inport
  Constant1 : Constant  Value=variable
  Product1 : Product
  q rounder16 : Subsystem  mask{q=nQ, range=maxRange}
      mask prompts: q "q value"; range "q range"
  out : Outport
  wires:
  q rounder16/1(out) -> Product1/1
  Constant1/1 -> q rounder16/1(in)
  Product1/1 -> out/1
  in/1 -> Product1/2

== system general_charger_2 (Jordans MacBook.lan's conflicted copy 2013-12-22)/Measurements/discrete low pass filter1/Cd(1) ==
  in : Inport
  Constant1 : Constant  Value=variable
  Product1 : Product
  q rounder16 : Subsystem  mask{q=nQ, range=maxRange}
      mask prompts: q "q value"; range "q range"
  out : Outport
  wires:
  q rounder16/1(out) -> Product1/1
  Constant1/1 -> q rounder16/1(in)
  Product1/1 -> out/1
  in/1 -> Product1/2

== system general_charger_2 (Jordans MacBook.lan's conflicted copy 2013-12-22)/Measurements/discrete low pass filter1/Cd(2) ==
  in : Inport
  Constant1 : Constant  Value=variable
  Product1 : Product
  q rounder16 : Subsystem  mask{q=nQ, range=maxRange}
      mask prompts: q "q value"; range "q range"
  out : Outport
  wires:
  q rounder16/1(out) -> Product1/1
  Constant1/1 -> q rounder16/1(in)
  Product1/1 -> out/1
  in/1 -> Product1/2

== system general_charger_2 (Jordans MacBook.lan's conflicted copy 2013-12-22)/Measurements/discrete low pass filter1/Cd(3) ==
  in : Inport
  Constant1 : Constant  Value=variable
  Product1 : Product
  q rounder16 : Subsystem  mask{q=nQ, range=maxRange}
      mask prompts: q "q value"; range "q range"
  out : Outport
  wires:
  q rounder16/1(out) -> Product1/1
  Constant1/1 -> q rounder16/1(in)
  Product1/1 -> out/1
  in/1 -> Product1/2

== system general_charger_2 (Jordans MacBook.lan's conflicted copy 2013-12-22)/Measurements/discrete low pass filter1/Dd ==
  in : Inport
  Constant1 : Constant  Value=variable
  Product1 : Product
  Scope1 : Scope  NumInputPorts=2
      settings: YMin=-5~-5  YMax=5~5
  q rounder16 : Subsystem  mask{q=nQ, range=maxRange}
      mask prompts: q "q value"; range "q range"
  out : Outport
  wires:
  q rounder16/1(out) -> Product1/1, Scope1/2
  Constant1/1 -> Scope1/1, q rounder16/1(in)
  Product1/1 -> out/1
  in/1 -> Product1/2

== system general_charger_2 (Jordans MacBook.lan's conflicted copy 2013-12-22)/Measurements/discrete low pass filter1/q rounder1 ==
  in : Inport
  Gain9 : Gain  Gain=2^-q
  Idealized ADC quantizer : simulink_extras/Additional Discrete/Idealized ADC quantizer  NumberOfConverterBits=32  Vmin=-range  Vmax=range  OutputDataType=double  OutputNegativeValues=on
  out : Outport
  wires:
  in/1 -> Idealized ADC quantizer/1
  Idealized ADC quantizer/1 -> Gain9/1
  Gain9/1 -> out/1

== system general_charger_2 (Jordans MacBook.lan's conflicted copy 2013-12-22)/Measurements/discrete low pass filter1/q rounder10 ==
  in : Inport
  Gain9 : Gain  Gain=2^-q
  Idealized ADC quantizer : simulink_extras/Additional Discrete/Idealized ADC quantizer  NumberOfConverterBits=32  Vmin=-range  Vmax=range  OutputDataType=double  OutputNegativeValues=on
  out : Outport
  wires:
  in/1 -> Idealized ADC quantizer/1
  Idealized ADC quantizer/1 -> Gain9/1
  Gain9/1 -> out/1

== system general_charger_2 (Jordans MacBook.lan's conflicted copy 2013-12-22)/Measurements/discrete low pass filter1/q rounder11 ==
  in : Inport
  Gain9 : Gain  Gain=2^-q
  Idealized ADC quantizer : simulink_extras/Additional Discrete/Idealized ADC quantizer  NumberOfConverterBits=32  Vmin=-range  Vmax=range  OutputDataType=double  OutputNegativeValues=on
  out : Outport
  wires:
  in/1 -> Idealized ADC quantizer/1
  Idealized ADC quantizer/1 -> Gain9/1
  Gain9/1 -> out/1

== system general_charger_2 (Jordans MacBook.lan's conflicted copy 2013-12-22)/Measurements/discrete low pass filter1/q rounder12 ==
  in : Inport
  Gain9 : Gain  Gain=2^-q
  Idealized ADC quantizer : simulink_extras/Additional Discrete/Idealized ADC quantizer  NumberOfConverterBits=32  Vmin=-range  Vmax=range  OutputDataType=double  OutputNegativeValues=on
  out : Outport
  wires:
  in/1 -> Idealized ADC quantizer/1
  Idealized ADC quantizer/1 -> Gain9/1
  Gain9/1 -> out/1

== system general_charger_2 (Jordans MacBook.lan's conflicted copy 2013-12-22)/Measurements/discrete low pass filter1/q rounder13 ==
  in : Inport
  Gain9 : Gain  Gain=2^-q
  Idealized ADC quantizer : simulink_extras/Additional Discrete/Idealized ADC quantizer  NumberOfConverterBits=32  Vmin=-range  Vmax=range  OutputDataType=double  OutputNegativeValues=on
  out : Outport
  wires:
  in/1 -> Idealized ADC quantizer/1
  Idealized ADC quantizer/1 -> Gain9/1
  Gain9/1 -> out/1

== system general_charger_2 (Jordans MacBook.lan's conflicted copy 2013-12-22)/Measurements/discrete low pass filter1/q rounder14 ==
  in : Inport
  Gain9 : Gain  Gain=2^-q
  Idealized ADC quantizer : simulink_extras/Additional Discrete/Idealized ADC quantizer  NumberOfConverterBits=32  Vmin=-range  Vmax=range  OutputDataType=double  OutputNegativeValues=on
  out : Outport
  wires:
  in/1 -> Idealized ADC quantizer/1
  Idealized ADC quantizer/1 -> Gain9/1
  Gain9/1 -> out/1

== system general_charger_2 (Jordans MacBook.lan's conflicted copy 2013-12-22)/Measurements/discrete low pass filter1/q rounder15 ==
  in : Inport
  Gain9 : Gain  Gain=2^-q
  Idealized ADC quantizer : simulink_extras/Additional Discrete/Idealized ADC quantizer  NumberOfConverterBits=32  Vmin=-range  Vmax=range  OutputDataType=double  OutputNegativeValues=on
  out : Outport
  wires:
  in/1 -> Idealized ADC quantizer/1
  Idealized ADC quantizer/1 -> Gain9/1
  Gain9/1 -> out/1

== system general_charger_2 (Jordans MacBook.lan's conflicted copy 2013-12-22)/Measurements/discrete low pass filter1/q rounder16 ==
  in : Inport
  Gain9 : Gain  Gain=2^-q
  Idealized ADC quantizer : simulink_extras/Additional Discrete/Idealized ADC quantizer  NumberOfConverterBits=32  Vmin=-range  Vmax=range  OutputDataType=double  OutputNegativeValues=on
  out : Outport
  wires:
  in/1 -> Idealized ADC quantizer/1
  Idealized ADC quantizer/1 -> Gain9/1
  Gain9/1 -> out/1

== system general_charger_2 (Jordans MacBook.lan's conflicted copy 2013-12-22)/Measurements/discrete low pass filter1/q rounder17 ==
  in : Inport
  Gain9 : Gain  Gain=2^-q
  Idealized ADC quantizer : simulink_extras/Additional Discrete/Idealized ADC quantizer  NumberOfConverterBits=32  Vmin=-range  Vmax=range  OutputDataType=double  OutputNegativeValues=on
  out : Outport
  wires:
  in/1 -> Idealized ADC quantizer/1
  Idealized ADC quantizer/1 -> Gain9/1
  Gain9/1 -> out/1

== system general_charger_2 (Jordans MacBook.lan's conflicted copy 2013-12-22)/Measurements/discrete low pass filter1/q rounder2 ==
  in : Inport
  Gain9 : Gain  Gain=2^-q
  Idealized ADC quantizer : simulink_extras/Additional Discrete/Idealized ADC quantizer  NumberOfConverterBits=32  Vmin=-range  Vmax=range  OutputDataType=double  OutputNegativeValues=on
  out : Outport
  wires:
  in/1 -> Idealized ADC quantizer/1
  Idealized ADC quantizer/1 -> Gain9/1
  Gain9/1 -> out/1

== system general_charger_2 (Jordans MacBook.lan's conflicted copy 2013-12-22)/Measurements/discrete low pass filter1/q rounder3 ==
  in : Inport
  Gain9 : Gain  Gain=2^-q
  Idealized ADC quantizer : simulink_extras/Additional Discrete/Idealized ADC quantizer  NumberOfConverterBits=32  Vmin=-range  Vmax=range  OutputDataType=double  OutputNegativeValues=on
  out : Outport
  wires:
  in/1 -> Idealized ADC quantizer/1
  Idealized ADC quantizer/1 -> Gain9/1
  Gain9/1 -> out/1

== system general_charger_2 (Jordans MacBook.lan's conflicted copy 2013-12-22)/Measurements/discrete low pass filter1/q rounder4 ==
  in : Inport
  Gain9 : Gain  Gain=2^-q
  Idealized ADC quantizer : simulink_extras/Additional Discrete/Idealized ADC quantizer  NumberOfConverterBits=32  Vmin=-range  Vmax=range  OutputDataType=double  OutputNegativeValues=on
  out : Outport
  wires:
  in/1 -> Idealized ADC quantizer/1
  Idealized ADC quantizer/1 -> Gain9/1
  Gain9/1 -> out/1

== system general_charger_2 (Jordans MacBook.lan's conflicted copy 2013-12-22)/Measurements/discrete low pass filter1/q rounder5 ==
  in : Inport
  Gain9 : Gain  Gain=2^-q
  Idealized ADC quantizer : simulink_extras/Additional Discrete/Idealized ADC quantizer  NumberOfConverterBits=32  Vmin=-range  Vmax=range  OutputDataType=double  OutputNegativeValues=on
  out : Outport
  wires:
  in/1 -> Idealized ADC quantizer/1
  Idealized ADC quantizer/1 -> Gain9/1
  Gain9/1 -> out/1

== system general_charger_2 (Jordans MacBook.lan's conflicted copy 2013-12-22)/Measurements/discrete low pass filter1/q rounder6 ==
  in : Inport
  Gain9 : Gain  Gain=2^-q
  Idealized ADC quantizer : simulink_extras/Additional Discrete/Idealized ADC quantizer  NumberOfConverterBits=32  Vmin=-range  Vmax=range  OutputDataType=double  OutputNegativeValues=on
  out : Outport
  wires:
  in/1 -> Idealized ADC quantizer/1
  Idealized ADC quantizer/1 -> Gain9/1
  Gain9/1 -> out/1

== system general_charger_2 (Jordans MacBook.lan's conflicted copy 2013-12-22)/Measurements/discrete low pass filter1/q rounder7 ==
  in : Inport
  Gain9 : Gain  Gain=2^-q
  Idealized ADC quantizer : simulink_extras/Additional Discrete/Idealized ADC quantizer  NumberOfConverterBits=32  Vmin=-range  Vmax=range  OutputDataType=double  OutputNegativeValues=on
  out : Outport
  wires:
  in/1 -> Idealized ADC quantizer/1
  Idealized ADC quantizer/1 -> Gain9/1
  Gain9/1 -> out/1

== system general_charger_2 (Jordans MacBook.lan's conflicted copy 2013-12-22)/Measurements/discrete low pass filter1/q rounder8 ==
  in : Inport
  Gain9 : Gain  Gain=2^-q
  Idealized ADC quantizer : simulink_extras/Additional Discrete/Idealized ADC quantizer  NumberOfConverterBits=32  Vmin=-range  Vmax=range  OutputDataType=double  OutputNegativeValues=on
  out : Outport
  wires:
  in/1 -> Idealized ADC quantizer/1
  Idealized ADC quantizer/1 -> Gain9/1
  Gain9/1 -> out/1

== system general_charger_2 (Jordans MacBook.lan's conflicted copy 2013-12-22)/Measurements/discrete low pass filter1/q rounder9 ==
  in : Inport
  Gain9 : Gain  Gain=2^-q
  Idealized ADC quantizer : simulink_extras/Additional Discrete/Idealized ADC quantizer  NumberOfConverterBits=32  Vmin=-range  Vmax=range  OutputDataType=double  OutputNegativeValues=on
  out : Outport
  wires:
  in/1 -> Idealized ADC quantizer/1
  Idealized ADC quantizer/1 -> Gain9/1
  Gain9/1 -> out/1

== system general_charger_2 (Jordans MacBook.lan's conflicted copy 2013-12-22)/control_stage/AC//DC Control/DQ Controller ==
  inputs : Inport
  AB-DQ Transform : Subsystem
  DQ Controller Submodule : Subsystem  mask{vdc=dc_volt, f=60, vdc_ki=dq_vdc_ki, vdc_kp=dq_vdc_kp, id_ki=dq_id_ki, id_kp=dq_id_kp, iq_ki=dq_iq_ki, iq_kp=dq_iq_kp, Ts=switch_Ts, L=Lin, R=Rin, turn_on=reactive_power_on}
      mask prompts: vdc "DC Voltage Reference"; f "Frequency (Hz)"; vdc_ki "Vdc Integral Gain"; vdc_kp "Vdc Proportional Gain"; id_ki "Id Integral Gain"; id_kp "Id  Proportional Gain"; iq_ki "Iq Integral Gain"; iq_kp "Iq Proportional Gain"; Ts "Sample Time"; L "Input Inductance (H)"; R "Input Resistance (ohms)"; turn_on "Reactive Power Control Turn on Time (s)"
  Demux : Demux  Outputs=3
  discrete low pass filter1 : Subsystem
      mask Display: disp('filter');
  v_cont : Outport
  tag scope: Id=global, Iq=global, Vd=global, Vq=global, Vwt=global
  wires:
  DQ Controller Submodule/1(Va) -> v_cont/1
  Demux/2 -> DQ Controller Submodule/1(Vdc)  "vdc"
  inputs/1 -> Demux/1
  Demux/1 -> discrete low pass filter1/1(filter in)  "vac"
  Demux/3 -> AB-DQ Transform/2(Ia)  "iac"
  AB-DQ Transform/2(Vq) -> [Vq]
  AB-DQ Transform/3(Id) -> [Id], DQ Controller Submodule/3(Id)
  AB-DQ Transform/4(Iq) -> [Iq], DQ Controller Submodule/4(Iq)
  AB-DQ Transform/5(theta) -> [Vwt], DQ Controller Submodule/5(Vwt)
  discrete low pass filter1/1(filter out) -> AB-DQ Transform/1(Va)
  AB-DQ Transform/1(Vd) -> DQ Controller Submodule/2(Vd), [Vd]
  [phi] -> AB-DQ Transform/3(phi)

== system general_charger_2 (Jordans MacBook.lan's conflicted copy 2013-12-22)/control_stage/AC//DC Control/Full Birdge IGBT drivers ==
  v_cont : Inport
  Add : Sum
  Add1 : Sum
  Constant1 : Constant  Value=1250
  Constant2 : Constant  Value=-1250
  Constant3 : Constant  Value=1250
  Constant4 : Constant  Value=1250
  Logical Operator : Logic  Operator=NOT  AllPortsSameDT=off  OutDataTypeStr=boolean
  Logical Operator1 : Logic  Operator=NOT  AllPortsSameDT=off  OutDataTypeStr=boolean
  Mux : Mux  Inputs=2
  Mux1 : Mux  Inputs=2
  Product2 : Product  RndMeth=Zero
  Product6 : Product  RndMeth=Zero
  Relational Operator : RelationalOperator  Operator=<=  OutDataTypeStr=boolean
  Relational Operator1 : RelationalOperator  Operator=<=  OutDataTypeStr=boolean
  Repeating Sequence : simulink/Sources/Repeating Sequence  rep_seq_t=[0 25e-6 50e-6]  rep_seq_y=[0 2500 0]
  Repeating Sequence2 : simulink/Sources/Repeating Sequence  rep_seq_t=[0 25e-6 50e-6]  rep_seq_y=[0 2500 0]
  Saturation : Saturate  UpperLimit=2500  LowerLimit=0
  Saturation1 : Saturate  UpperLimit=2500  LowerLimit=0
  Scope1 : Scope  NumInputPorts=2
      settings: TimeRange=0.5  YMin=-5~-5  YMax=5~5  SaveName=vcontrol_  MaxDataPoints=50000
  Scope2 : Scope
      settings: SaveName=ScopeData5
  Scope3 : Scope
      settings: SaveName=ScopeData10
  Scope4 : Scope  NumInputPorts=2
      settings: TimeRange=0.5  YMin=-5~-5  YMax=5~5  SaveName=vcontrol_1  MaxDataPoints=50000
  tag scope: A=global, B=global, C=global, D=global
  wires:
  v_cont/1 -> Product2/2, Product6/2
  Logical Operator1/1 -> [B]
  Logical Operator/1 -> [D]
  Repeating Sequence2/1 -> Relational Operator1/2, Mux/1, Scope3/1
  Relational Operator1/1 -> [C], Logical Operator/1, Scope4/2
  Mux1/1 -> Scope1/1
  Mux/1 -> Scope4/1
  Constant2/1 -> Product2/1
  Repeating Sequence/1 -> Relational Operator/2, Mux1/1
  Relational Operator/1 -> [A], Scope1/2, Logical Operator1/1
  Constant3/1 -> Product6/1
  Saturation/1 -> Relational Operator/1, Mux1/2
  Saturation1/1 -> Relational Operator1/1, Mux/2
  Product6/1 -> Add/1
  Add/1 -> Saturation/1
  Product2/1 -> Add1/2
  Constant1/1 -> Add1/1
  Add1/1 -> Scope2/1, Saturation1/1
  Constant4/1 -> Add/2
